simulink model "untitled"  (R2020a)
settings: Solver=FixedStepAuto  StartTime=0.0  StopTime=10.0  FixedStep=0.00001  RelTol=1e-3
values from neighbouring files (symbols this model uses):
  fref = 100    [Untitled.m]
  L = [0.01 0 0 0 0;0 0.01 0 0 0;0 0 0.01 0 0;0 0 0 0.01 0;0 0 0 0 0.01]    [Untitled.m]
  R = [1 0 0 0 0;0 1 0 0 0;0 0 1 0 0;0 0 0 1 0;0 0 0 0 1]    [Untitled.m]
  T = [4 -1 -1 -1 -1;-1 4 -1 -1 -1;-1 -1 4 -1 -1;-1 -1 -1 4 -1;-1 -1 -1 -1 4]    [Untitled.m]
  vdc = 300    [Untitled.m]
settings Model: Creator=ABO-CHIFA  LastModifiedBy=ABO-CHIFA

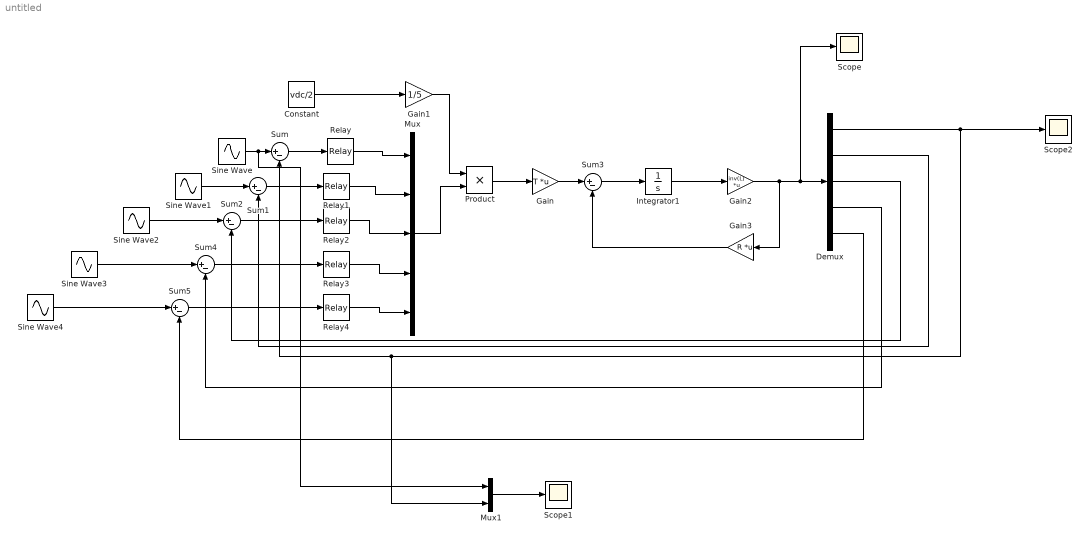
== system untitled ==
  Constant : Constant  Value=vdc/2
  Demux : Demux  Outputs=5
  Gain : Gain  Gain=T  Multiplication=Matrix(K*u)
  Gain1 : Gain  Gain=1/5
  Gain2 : Gain  Gain=inv(L)  Multiplication=Matrix(K*u)
  Gain3 : Gain  Gain=R  Multiplication=Matrix(K*u)
  Integrator1 : Integrator
  Mux : Mux  Inputs=5
  Mux1 : Mux  Inputs=2
  Product : Product
  Relay{,1..4} (5 alike) : Relay  OnSwitchValue=0.5  OffSwitchValue=-0.5  OffOutputValue=-1
  Scope : Scope
  Scope1 : Scope
  Scope2 : Scope
  Sine Wave : Sin  Amplitude=20  Frequency=2*pi*fref  SampleTime=0
  Sine Wave1 : Sin  Amplitude=20  Frequency=2*pi*fref  Phase=2*pi/5  SampleTime=0
  Sine Wave2 : Sin  Amplitude=20  Frequency=2*pi*fref  Phase=4*pi/5  SampleTime=0
  Sine Wave3 : Sin  Amplitude=20  Frequency=2*pi*fref  Phase=6*pi/5  SampleTime=0
  Sine Wave4 : Sin  Amplitude=20  Frequency=2*pi*fref  Phase=8*pi/5  SampleTime=0
  Sum{,1..5} (6 alike) : Sum  Inputs=|+-
  wires:
  Mux/1 -> Product/2
  Gain1/1 -> Product/1
  Constant/1 -> Gain1/1
  Relay/1 -> Mux/1
  Relay1/1 -> Mux/2
  Relay2/1 -> Mux/3
  Sum/1 -> Relay/1
  Sum1/1 -> Relay1/1
  Sine Wave1/1 -> Sum1/1
  Sum2/1 -> Relay2/1
  Sine Wave2/1 -> Sum2/1
  Gain/1 -> Sum3/1
  Sum3/1 -> Integrator1/1
  Integrator1/1 -> Gain2/1
  Gain3/1 -> Sum3/2
  Gain2/1 -> Gain3/1, Scope/1, Demux/1
  Sine Wave3/1 -> Sum4/1
  Sum4/1 -> Relay3/1
  Relay3/1 -> Mux/4
  Sum5/1 -> Relay4/1
  Sine Wave4/1 -> Sum5/1
  Relay4/1 -> Mux/5
  Demux/1 -> Mux1/2, Sum/2, Scope2/1
  Demux/2 -> Sum1/2
  Demux/3 -> Sum2/2
  Demux/4 -> Sum4/2
  Demux/5 -> Sum5/2
  Mux1/1 -> Scope1/1
  Sine Wave/1 -> Mux1/1, Sum/1
  Product/1 -> Gain/1
